simulink model "Plant_1_2_modified"  (R2024b)
settings: Solver=VariableStepAuto  StartTime=0.0  StopTime=2  RelTol=1e-3
undefined symbols (not defined in the file or in its folder): A, B
libraries: slpidlib x2
settings Model: Creator=Sez26  LastModifiedBy=herra

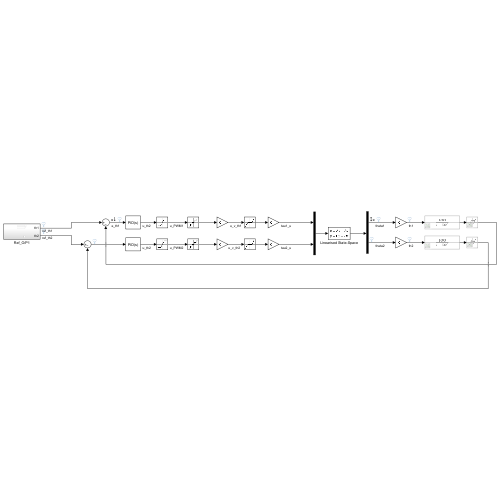
[thumbnail: Simulink's stored preview of the top-level diagram]
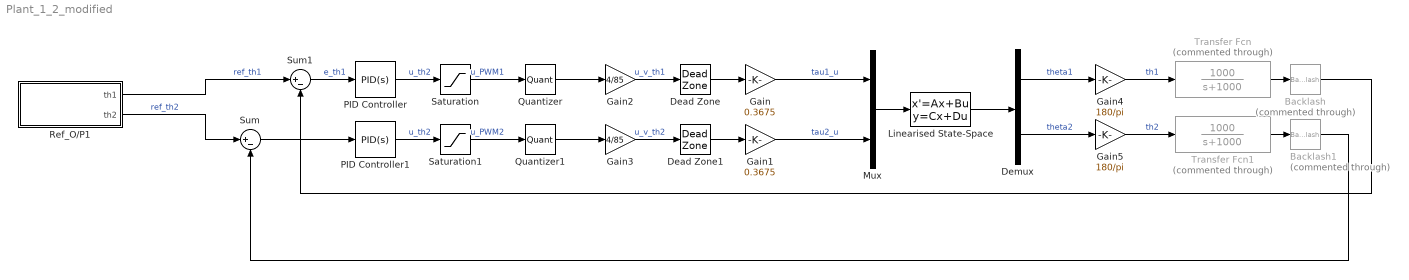
== system Plant_1_2_modified ==
  Backlash : Backlash  Commented=through  BacklashWidth=3
  Backlash1 : Backlash  Commented=through  BacklashWidth=3
  Dead Zone : DeadZone  LowerValue=-2.1  UpperValue=2.1
  Dead Zone1 : DeadZone  LowerValue=-2.1  UpperValue=2.1
  Demux : Demux  Outputs=2
  Gain : Gain  Gain=0.3675
  Gain1 : Gain  Gain=0.3675
  Gain2 : Gain  Gain=4/85
  Gain3 : Gain  Gain=4/85
  Gain4 : Gain  Gain=180/pi
  Gain5 : Gain  Gain=180/pi
  Linearised State-Space : StateSpace  A=A  B=B  C=[1 0 0 0; 0 1 0 0]  D=[0 0; 0 0]  InitialCondition=0
  Mux : Mux  Inputs=2
  PID Controller : slpidlib/PID Controller  Controller=PID  Form=Parallel  TimeDomain=Continuous-time  UseExternalTs=off  SampleTime=-1  IntegratorMethod=Forward Euler  FilterMethod=Forward Euler  ControllerParametersSource=internal  P=1788.95104092049  I=1998.5357721302  UseKiTs=off  D=13.6992193813271  UseExternalDerivativeSource=off  N=14717.681597445  UseFilter=on  TunerSelectOption=Transfer Function Based (PID Tuner App)  InitialConditionSource=internal  InitialConditionForIntegrator=0  InitialConditionForFilter=0  DifferentiatorICPrevScaledInput=0  ExternalReset=none  TrackingMode=off  Kt=1  LimitOutput=off  SatLimitsSource=internal  UpperSaturationLimit=inf  LowerSaturationLimit=-inf  LinearizeAsGain=on  AntiWindupMode=none  Kb=1  LimitIntegrator=off  UpperIntegratorSaturationLimit=inf  LowerIntegratorSaturationLimit=-inf  POutMin=[]  POutMax=[]  IOutMin=[]  IOutMax=[]  DOutMin=[]  DOutMax=[]  NOutMin=[]  NOutMax=[]  SumOutMin=[]  SumOutMax=[]  SaturationOutMin=[]  SaturationOutMax=[]  PParamMin=[]  PParamMax=[]  IParamMin=[]  IParamMax=[]  DParamMin=[]  DParamMax=[]  NParamMin=[]  NParamMax=[]  KbParamMin=[]  KbParamMax=[]  KtParamMin=[]  KtParamMax=[]  KbOutMin=[]  KbOutMax=[]  KtOutMin=[]  KtOutMax=[]  IntegratorOutMin=[]  IntegratorOutMax=[]  FilterOutMin=[]  FilterOutMax=[]  SumI1OutMin=[]  SumI1OutMax=[]  SumI2OutMin=[]  SumI2OutMax=[]  SumI3OutMin=[]  SumI3OutMax=[]  SumI4OutMin=[]  SumI4OutMax=[]  SumDOutMin=[]  SumDOutMax=[]  DifferentiatorOutMin=[]  DifferentiatorOutMax=[]  FilterDiffOutCoefMin=[]  FilterDiffOutCoefMax=[]  ReciprocalOutMin=[]  ReciprocalOutMax=[]  SumDenOutMin=[]  SumDenOutMax=[]  SumNumOutMin=[]  SumNumOutMax=[]  DivideOutMin=[]  DivideOutMax=[]  UdiffTsProdOutMin=[]  UdiffTsProdOutMax=[]  NTsProdOutMin=[]  NTsProdOutMax=[]  UintegralTsProdOutMin=[]  UintegralTsProdOutMax=[]  UngainTsProdOutMin=[]  UngainTsProdOutMax=[]  ClampingZeroOutDataTypeStr=Inherit: Inherit via back propagation  ClampingZeroOutMin=[]  ClampingZeroOutMax=[]  FilterDenConstantOutDataTypeStr=Inherit: Inherit via back propagation  FilterDenConstantOutMin=[]  FilterDenConstantOutMax=[]  PCopyOutDataTypeStr=Inherit: Inherit via back propagation  PCopyOutMin=[]  PCopyOutMax=[]  NCopyOutDataTypeStr=Inherit: Inherit via back propagation  NCopyOutMin=[]  NCopyOutMax=[]  IntegratorContinuousStateAttributes=''  IntegratorStateMustResolveToSignalObject=off  IntegratorRTWStateStorageClass=Auto  FilterContinuousStateAttributes=''  FilterStateMustResolveToSignalObject=off  FilterRTWStateStorageClass=Auto  ParallelPVariant=InternalParameters  IdealPVariant=Disabled  IVariant=InternalParameters  DVariant=InternalParameters  IntegratorVariant=Continuous  SatVariant=Disabled  AWVariant=Passthrough  PCopyVariant=Disabled  TRVariant=Disabled  FdbkBlocksVariant=Forward  IdealPFdbkVariant=Disabled  SatFdbkVariant=Disabled  DerivativeFilterVariant=ContFilter  NVariant=InternalParameters  NCopyVariant=Disabled  FilterICVariant=InternalICsFilter  IntegratorICVariant=InternalICs  ExternalResetVariant=Disabled  TRSumVariant=Passthrough  SumFdbkVariant=Disabled  SumVariant=Sum_PID  TsampFilterVariant=InternalTs  TsampNgainVariant=Passthrough  TsampIntegralVariant=Disabled_SignalSpec  ExternalSaturationOutDataTypeStr=Inherit: Same as second input  DerivativeSourceVariant=ErrorSignal  PreIntVariant=InternalPreInt
  PID Controller1 : slpidlib/PID Controller  Controller=PID  Form=Parallel  TimeDomain=Continuous-time  UseExternalTs=off  SampleTime=-1  IntegratorMethod=Forward Euler  FilterMethod=Forward Euler  ControllerParametersSource=internal  P=1789  I=1999  UseKiTs=off  D=13.7  UseExternalDerivativeSource=off  N=14720  UseFilter=on  TunerSelectOption=Transfer Function Based (PID Tuner App)  InitialConditionSource=internal  InitialConditionForIntegrator=0  InitialConditionForFilter=0  DifferentiatorICPrevScaledInput=0  ExternalReset=none  TrackingMode=off  Kt=1  LimitOutput=off  SatLimitsSource=internal  UpperSaturationLimit=inf  LowerSaturationLimit=-inf  LinearizeAsGain=on  AntiWindupMode=none  Kb=1  LimitIntegrator=off  UpperIntegratorSaturationLimit=inf  LowerIntegratorSaturationLimit=-inf  POutMin=[]  POutMax=[]  IOutMin=[]  IOutMax=[]  DOutMin=[]  DOutMax=[]  NOutMin=[]  NOutMax=[]  SumOutMin=[]  SumOutMax=[]  SaturationOutMin=[]  SaturationOutMax=[]  PParamMin=[]  PParamMax=[]  IParamMin=[]  IParamMax=[]  DParamMin=[]  DParamMax=[]  NParamMin=[]  NParamMax=[]  KbParamMin=[]  KbParamMax=[]  KtParamMin=[]  KtParamMax=[]  KbOutMin=[]  KbOutMax=[]  KtOutMin=[]  KtOutMax=[]  IntegratorOutMin=[]  IntegratorOutMax=[]  FilterOutMin=[]  FilterOutMax=[]  SumI1OutMin=[]  SumI1OutMax=[]  SumI2OutMin=[]  SumI2OutMax=[]  SumI3OutMin=[]  SumI3OutMax=[]  SumI4OutMin=[]  SumI4OutMax=[]  SumDOutMin=[]  SumDOutMax=[]  DifferentiatorOutMin=[]  DifferentiatorOutMax=[]  FilterDiffOutCoefMin=[]  FilterDiffOutCoefMax=[]  ReciprocalOutMin=[]  ReciprocalOutMax=[]  SumDenOutMin=[]  SumDenOutMax=[]  SumNumOutMin=[]  SumNumOutMax=[]  DivideOutMin=[]  DivideOutMax=[]  UdiffTsProdOutMin=[]  UdiffTsProdOutMax=[]  NTsProdOutMin=[]  NTsProdOutMax=[]  UintegralTsProdOutMin=[]  UintegralTsProdOutMax=[]  UngainTsProdOutMin=[]  UngainTsProdOutMax=[]  ClampingZeroOutDataTypeStr=Inherit: Inherit via back propagation  ClampingZeroOutMin=[]  ClampingZeroOutMax=[]  FilterDenConstantOutDataTypeStr=Inherit: Inherit via back propagation  FilterDenConstantOutMin=[]  FilterDenConstantOutMax=[]  PCopyOutDataTypeStr=Inherit: Inherit via back propagation  PCopyOutMin=[]  PCopyOutMax=[]  NCopyOutDataTypeStr=Inherit: Inherit via back propagation  NCopyOutMin=[]  NCopyOutMax=[]  IntegratorContinuousStateAttributes=''  IntegratorStateMustResolveToSignalObject=off  IntegratorRTWStateStorageClass=Auto  FilterContinuousStateAttributes=''  FilterStateMustResolveToSignalObject=off  FilterRTWStateStorageClass=Auto  ParallelPVariant=InternalParameters  IdealPVariant=Disabled  IVariant=InternalParameters  DVariant=InternalParameters  IntegratorVariant=Continuous  SatVariant=Disabled  AWVariant=Passthrough  PCopyVariant=Disabled  TRVariant=Disabled  FdbkBlocksVariant=Forward  IdealPFdbkVariant=Disabled  SatFdbkVariant=Disabled  DerivativeFilterVariant=ContFilter  NVariant=InternalParameters  NCopyVariant=Disabled  FilterICVariant=InternalICsFilter  IntegratorICVariant=InternalICs  ExternalResetVariant=Disabled  TRSumVariant=Passthrough  SumFdbkVariant=Disabled  SumVariant=Sum_PID  TsampFilterVariant=InternalTs  TsampNgainVariant=Passthrough  TsampIntegralVariant=Disabled_SignalSpec  ExternalSaturationOutDataTypeStr=Inherit: Same as second input  DerivativeSourceVariant=ErrorSignal  PreIntVariant=InternalPreInt
  Quantizer : Quantizer  QuantizationInterval=1
  Quantizer1 : Quantizer  QuantizationInterval=1
  Ref_O/P1 : Subsystem
  Saturation : Saturate  UpperLimit=255  LowerLimit=-255
  Saturation1 : Saturate  UpperLimit=255  LowerLimit=-255
  Sum : Sum  Inputs=|+-
  Sum1 : Sum  Inputs=|+-
  Transfer Fcn : TransferFcn  Commented=through  Numerator=[1000]  Denominator=[1 1000]
  Transfer Fcn1 : TransferFcn  Commented=through  Numerator=[1000]  Denominator=[1 1000]
  wires:
  Linearised State-Space/1 -> Demux/1
  Demux/1 -> Gain4/1  "theta1"
  Demux/2 -> Gain5/1  "theta2"
  Sum/1 -> PID Controller1/1
  Sum1/1 -> PID Controller/1  "e_th1"
  Gain3/1 -> Dead Zone1/1  "u_v_th2"
  PID Controller/1 -> Saturation/1  "u_th2"
  Quantizer1/1 -> Gain3/1
  PID Controller1/1 -> Saturation1/1  "u_th2"
  Saturation/1 -> Quantizer/1  "u_PWM1"
  Dead Zone/1 -> Gain/1
  Quantizer/1 -> Gain2/1
  Gain2/1 -> Dead Zone/1  "u_v_th1"
  Dead Zone1/1 -> Gain1/1
  Saturation1/1 -> Quantizer1/1  "u_PWM2"
  Ref_O/P1/1(th1) -> Sum1/1  "ref_th1"
  Ref_O/P1/2(th2) -> Sum/1  "ref_th2"
  Mux/1 -> Linearised State-Space/1
  Gain/1 -> Mux/1  "tau1_u"
  Gain1/1 -> Mux/2  "tau2_u"
  Gain5/1 -> Transfer Fcn1/1  "th2"
  Gain4/1 -> Transfer Fcn/1  "th1"
  Transfer Fcn/1 -> Backlash/1
  Transfer Fcn1/1 -> Backlash1/1
  Backlash/1 -> Sum1/2
  Backlash1/1 -> Sum/2

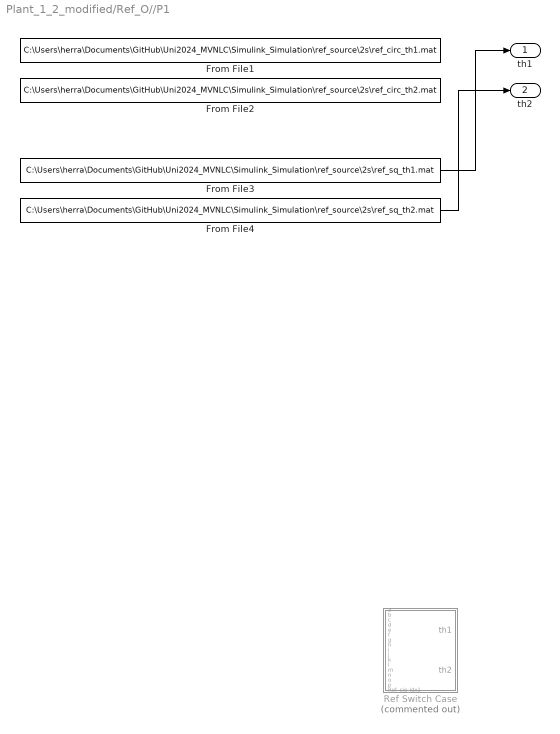
== system Plant_1_2_modified/Ref_O//P1 ==
  From File1 : FromFile  FileName=C:\Users\herra\Documents\GitHub\Uni2024_MVNLC\Simulink_Simulation\ref_source\2s\ref_circ_th1.mat  SampleTime=0
  From File2 : FromFile  FileName=C:\Users\herra\Documents\GitHub\Uni2024_MVNLC\Simulink_Simulation\ref_source\2s\ref_circ_th2.mat  SampleTime=0
  From File3 : FromFile  FileName=C:\Users\herra\Documents\GitHub\Uni2024_MVNLC\Simulink_Simulation\ref_source\2s\ref_sq_th1.mat  SampleTime=0
  From File4 : FromFile  FileName=C:\Users\herra\Documents\GitHub\Uni2024_MVNLC\Simulink_Simulation\ref_source\2s\ref_sq_th2.mat  SampleTime=0
  Ref Switch Case : MATLAB Function  Commented=on  TreatAsAtomicUnit=on
  th1 : Outport
  th2 : Outport  Port=2
  wires:
  From File3/1 -> th1/1
  From File4/1 -> th2/1

== matlab function Plant_1_2_modified/Ref_O//P1/Ref Switch Case ==
  data: Ref_sig_idx parameter; a input; b input; c input; d input; e input; f input; g input; h input; i input; j input; k input; l input; m input; n input; o input; p input; Ref_sig_idx1 input; th1 output; th2 output
function [th1, th2] = ref_switch(Ref_sig_idx, a, b, c, d, e, f, g, h, i, j, k, l, m, n, o, p, Ref_sig_idx1)
    if Ref_sig_idx == 0
        % circ base
        th1 = a;
        th2 = b;
    elseif Ref_sig_idx == 1
        % sq base
        th1 = c;
        th2 = d;
    elseif Ref_sig_idx == 2
        % tri base
        th1 = e;
        th2 = f;
    end
    if Ref_sig_idx == 3
        % circ b spline
        th1 = g;
        th2 = h;
    elseif Ref_sig_idx == 4
        % sq b spline
        th1 = i;
        th2 = j;
    elseif Ref_sig_idx == 5
        % tri b spline
        th1 = k;
        th2 = l;
    end
    if Ref_sig_idx == 6
        % sq corner sf
        th1 = m;
        th2 = n;
    elseif Ref_sig_idx == 7
        % tri corner sf
        th1 = o;
        th2 = p;
    else
        % invalid reference choice
        disp('Error invalid reference choice')
        th1 = 0;
        th2 = 0;
    end
